simulink library "csc_lac_landing_acceleration_command_mtv_lib"  (R2014b)
settings: Solver=ode45  StartTime=0.0  StopTime=10.0  RelTol=1e-3
undefined symbols (not defined in the file or in its folder): csc_gdn_dt, lac_accel_available_init, lac_coarse_acs_thrust_available, lac_main_biprop_thrust_available, lac_monoprop_coarse_transition_alt
libraries: util_common_lib x4, simulink x1, util_info_lib x1, csc_ltg_landing_terminal_guidance_mtv_lib x1, csu_lat_landing_approach_targeting_lib x1, csu_lpc_landing_pre_coast_lib x1
settings Model: Creator=escrane  LastModifiedBy=tgorton

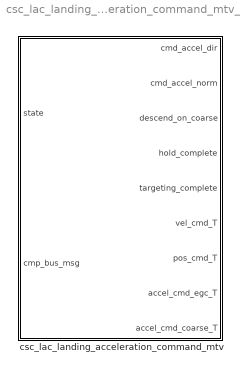
== system csc_lac_landing_acceleration_command_mtv_lib ==
  csc_lac_landing_acceleration_command_mtv : Subsystem

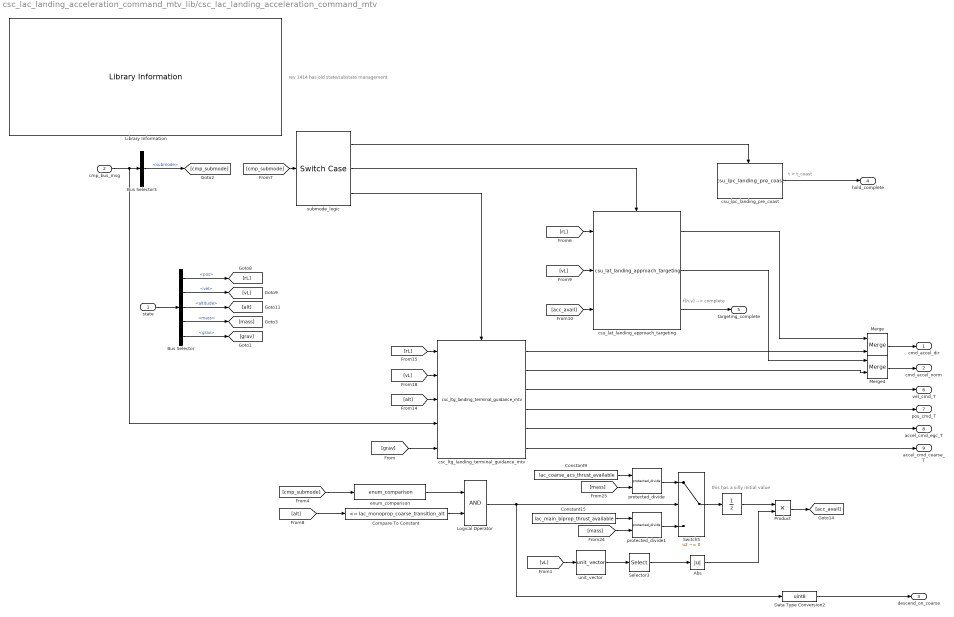
== system csc_lac_landing_acceleration_command_mtv_lib/csc_lac_landing_acceleration_command_mtv ==
  note: this has a silly initial value
  note: t > t_coast
  note: f(h,v) --> complete
  note: rev 1414 has old state/substate management
  state : Inport
  cmp_bus_msg : Inport  Port=2
  " " : UnitDelay  InitialCondition=lac_accel_available_init  SampleTime=csc_gdn_dt
  Abs : Abs
  Bus Selector : BusSelector  OutputSignals=pos,vel,altitude,mass,grav
  Bus Selector3 : BusSelector  OutputSignals=submode
  Compare To Constant : simulink/Logic and Bit Operations/Compare To Constant  relop=<=  const=lac_monoprop_coarse_transition_alt  OutDataTypeStr=boolean
  Constant15 : Constant  Value=lac_main_biprop_thrust_available
  Constant9 : Constant  Value=lac_coarse_acs_thrust_available
  Data Type Conversion2 : DataTypeConversion  OutDataTypeStr=uint8
  Library Information : util_info_lib/Library Information  owner='NONE'
  Logical Operator : Logic  AllPortsSameDT=off  OutDataTypeStr=boolean
  Merge : Merge  InitialOutput=[-1 0 0]'
  Merge4 : Merge  InitialOutput=0
  Product : Product
  Selector3 : Selector  InputPortWidth=3  Indices=[3]
  Switch5 : Switch  Criteria=u2 ~= 0
  csc_ltg_landing_terminal_guidance_mtv : csc_ltg_landing_terminal_guidance_mtv_lib/csc_ltg_landing_terminal_guidance_mtv
  csu_lat_landing_approach_targeting : csu_lat_landing_approach_targeting_lib/csu_lat_landing_approach_targeting
  csu_lpc_landing_pre_coast : csu_lpc_landing_pre_coast_lib/csu_lpc_landing_pre_coast
  enum_comparison : util_common_lib/enum_comparison  comparison_type===
  protected_divide : util_common_lib/protected_divide  fault_value=0  tolerance=eps
  protected_divide1 : util_common_lib/protected_divide  fault_value=0  tolerance=eps
  submode_logic : SwitchCase  CaseConditions={uint8(enum_submode.landing_hold), uint8(enum_submode.landing_targeting), uint8(enum_submode.landing_terminal)}  ShowDefaultCase=off
  unit_vector : util_common_lib/unit_vector  SystemSampleTime=-1
  cmd_accel_dir : Outport
  cmd_accel_norm : Outport  Port=2
  descend_on_coarse : Outport  Port=3  InitialOutput=1
  hold_complete : Outport  Port=4
  targeting_complete : Outport  Port=5
  vel_cmd_T : Outport  Port=6
  pos_cmd_T : Outport  Port=7
  accel_cmd_egc_T : Outport  Port=8
  accel_cmd_coarse_T : Outport  Port=9
  wires:
  [grav] -> csc_ltg_landing_terminal_guidance_mtv/5
  Bus Selector/5 -> [grav]  "<grav>"
  csc_ltg_landing_terminal_guidance_mtv/6 -> accel_cmd_coarse_T/1
  csc_ltg_landing_terminal_guidance_mtv/5 -> accel_cmd_egc_T/1
  csc_ltg_landing_terminal_guidance_mtv/1 -> Merge/2
  csc_ltg_landing_terminal_guidance_mtv/2 -> Merge4/2
  Merge/1 -> cmd_accel_dir/1
  Merge4/1 -> cmd_accel_norm/1
  csu_lat_landing_approach_targeting/1 -> Merge/1
  csu_lat_landing_approach_targeting/2 -> Merge4/1
  csc_ltg_landing_terminal_guidance_mtv/4 -> pos_cmd_T/1
  csc_ltg_landing_terminal_guidance_mtv/3 -> vel_cmd_T/1
  Bus Selector/1 -> [rL]  "<pos>"
  submode_logic/3 -> csc_ltg_landing_terminal_guidance_mtv/Action
  Constant15/1 -> protected_divide1/1
  Constant9/1 -> protected_divide/1
  csu_lat_landing_approach_targeting/3 -> targeting_complete/1
  Bus Selector/4 -> [mass]  "<mass>"
  [cmp_submode] -> submode_logic/1
  Bus Selector3/1 -> [cmp_submode]  "<submode>"
  csu_lpc_landing_pre_coast/1 -> hold_complete/1
  Compare To Constant/1 -> Logical Operator/2
  enum_comparison/1 -> Logical Operator/1
  [cmp_submode] -> enum_comparison/1
  submode_logic/2 -> csu_lat_landing_approach_targeting/Action
  submode_logic/1 -> csu_lpc_landing_pre_coast/Action
  [acc_avail] -> csu_lat_landing_approach_targeting/3
  [vL] -> csu_lat_landing_approach_targeting/2
  [rL] -> csu_lat_landing_approach_targeting/1
  state/1 -> Bus Selector/1
  [rL] -> csc_ltg_landing_terminal_guidance_mtv/1
  [vL] -> csc_ltg_landing_terminal_guidance_mtv/2
  Bus Selector/3 -> [alt]  "<altitude>"
  Bus Selector/2 -> [vL]  "<vel>"
  Logical Operator/1 -> Switch5/2, Data Type Conversion2/1
  Switch5/1 -> " "/1
  [mass] -> protected_divide/2
  [mass] -> protected_divide1/2
  protected_divide1/1 -> Switch5/3
  protected_divide/1 -> Switch5/1
  Data Type Conversion2/1 -> descend_on_coarse/1
  cmp_bus_msg/1 -> csc_ltg_landing_terminal_guidance_mtv/4, Bus Selector3/1
  [alt] -> csc_ltg_landing_terminal_guidance_mtv/3
  [alt] -> Compare To Constant/1
  unit_vector/1 -> Selector3/1
  Selector3/1 -> Abs/1
  " "/1 -> Product/1
  [vL] -> unit_vector/1
  Product/1 -> [acc_avail]
  Abs/1 -> Product/2
